simulink model "vllms_8_tap"  (R2021a)
settings: Solver=VariableStepAuto  StartTime=0.0  StopTime=4000  RelTol=1e-3
undefined symbols (not defined in the file): LeakyFactorCalc
libraries: dspsrcs4 x4, dspstat3 x4, dspmathops x2
settings Model: Creator=HP  LastModifiedBy=HP

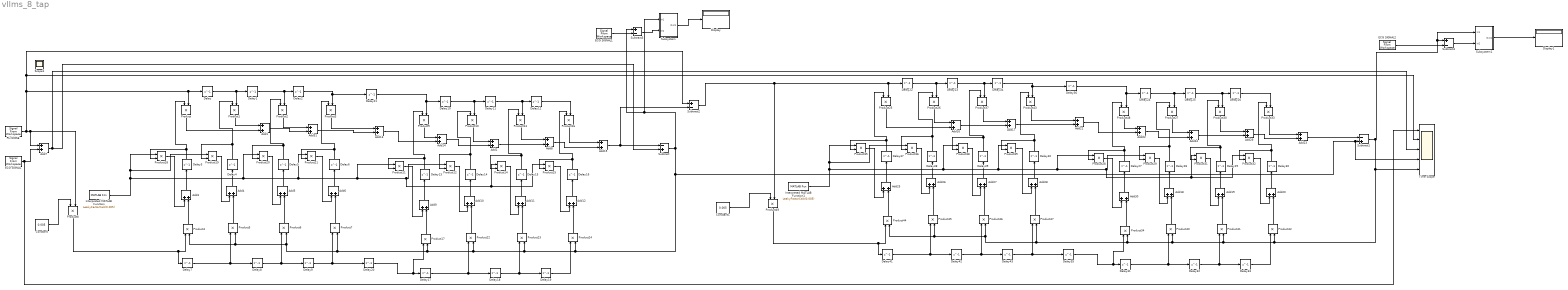
== system vllms_8_tap ==
  Add{1..31} (31 alike) : Sum
  Constant : Constant  Value=0.005
  Constant1 : Constant  Value=0.005
  Delay{,1..43} (44 alike) : Delay  DelayLength=1  InitialCondition=0
  Display : Display
  Display1 : Display
  ECG SIGNAL : dspsrcs4/Signal From Workspace  X=m1  Ts=1  nsamps=1  OutputAfterFinalValue=Setting to zero  ignoreOrWarnInputAndFrameLengths=off  OutputFrames=off
  ECG SIGNAL1 : dspsrcs4/Signal From Workspace  X=m1  Ts=1  nsamps=1  OutputAfterFinalValue=Setting to zero  ignoreOrWarnInputAndFrameLengths=off  OutputFrames=off
  ECG SIGNAL2 : dspsrcs4/Signal From Workspace  X=m1  Ts=1  nsamps=1  OutputAfterFinalValue=Setting to zero  ignoreOrWarnInputAndFrameLengths=off  OutputFrames=off
  Interpreted MATLAB Function : MATLABFcn  MATLABFcn=LeakyFactorCalc(0.005)
  Interpreted MATLAB Function1 : MATLABFcn  MATLABFcn=LeakyFactorCalc(0.005)
  PLI NOISE : dspsrcs4/Signal From Workspace  X=x1  Ts=1  nsamps=1  OutputAfterFinalValue=Setting to zero  ignoreOrWarnInputAndFrameLengths=off  OutputFrames=off
  Product{,1..49} (50 alike) : Product
  Subsystem : Subsystem
  Subsystem1 : Subsystem
  Subtract : Sum  Inputs=-+
  Subtract1 : Sum  Inputs=-+
  Subtract2 : Sum  Inputs=+-
  Subtract3 : Sum  Inputs=+-
  Subtract4 : Sum  Inputs=+-
  Time Scope : Scope  NumInputPorts=5
  Scope1 : Scope
  wires:
  Product7/1 -> Add6/2
  Delay6/1 -> Product21/2, Product3/1
  Delay1/1 -> Product2/2, Delay2/1
  PLI NOISE/1 -> Subtract2/1, Time Scope/2, Product/2, Delay/1, Product8/2, Add7/1
  Add4/1 -> Delay4/1
  Delay5/1 -> Product20/2, Product2/1
  Product5/1 -> Add4/2
  Product19/1 -> Add4/1
  Add5/1 -> Delay5/1
  Add6/1 -> Delay6/1
  Delay7/1 -> Delay8/1, Product5/1
  Product8/1 -> Product4/1, Delay7/1
  Delay8/1 -> Delay9/1, Product6/1
  Add3/1 -> Delay3/1
  Delay4/1 -> Product19/2, Product1/1
  Product4/1 -> Add3/2
  Product6/1 -> Add5/2
  Delay3/1 -> Product/1, Product18/2
  Product21/1 -> Add6/1
  Delay/1 -> Product1/2, Delay1/1
  Product20/1 -> Add5/1
  Product18/1 -> Add3/1
  Constant/1 -> Product8/1
  Product17/1 -> Add9/2
  Add9/1 -> Delay13/1
  Delay18/1 -> Delay19/1, Product23/1
  Delay11/1 -> Product13/2, Delay12/1
  Product24/1 -> Add12/2
  Interpreted MATLAB Function/1 -> Product20/1, Product21/1, Product14/1, Product15/1, Product12/1, Product11/1, Product19/1, Product18/1
  Add10/1 -> Delay14/1
  Product23/1 -> Add11/2
  Delay17/1 -> Delay18/1, Product22/1
  Delay12/1 -> Product16/2
  Product13/1 -> Add8/1
  Add12/1 -> Delay16/1
  Add2/1 -> Add8/2
  Add11/1 -> Delay15/1
  Delay9/1 -> Delay20/1, Product7/1
  Product12/1 -> Add10/1
  Product22/1 -> Add10/2
  Delay15/1 -> Product14/2, Product13/1
  Delay19/1 -> Product24/1
  Delay16/1 -> Product15/2, Product16/1
  Delay13/1 -> Product9/1, Product11/2
  Product15/1 -> Add12/1
  Product11/1 -> Add9/1
  Delay10/1 -> Product10/2, Delay11/1
  Delay14/1 -> Product12/2, Product10/1
  Product14/1 -> Add11/1
  Product10/1 -> Add2/1
  Delay2/1 -> Delay21/1, Product3/2
  Product9/1 -> Add14/1
  Add13/1 -> Add14/2
  Add14/1 -> Add2/2
  Add15/1 -> Subtract2/2, Subtract/1
  Product16/1 -> Add15/1
  Add8/1 -> Add15/2
  Delay20/1 -> Product17/1, Delay17/1
  Delay21/1 -> Product9/2, Delay10/1
  Add7/1 -> Time Scope/3, Subtract/2
  Add25/1 -> Delay37/1
  Product35/1 -> Add25/1
  Delay25/1 -> Product30/2, Delay26/1
  Product46/1 -> Add27/2
  Delay38/1 -> Product36/2, Product26/1
  Delay42/1 -> Delay43/1, Product46/1
  Product44/1 -> Add25/2
  Product43/1 -> Add21/1
  Delay28/1 -> Product29/2, Product27/1
  Delay29/1 -> Product31/2, Product30/1
  Subtract/1 -> Subsystem/1(In1), Subtract3/1, Time Scope/4, Subtract1/2, Product24/2, Product23/2, Product22/2, Product17/2, Product7/2, Product5/2, Product4/2, Product6/2
  Add26/1 -> Delay38/1
  Add29/1 -> Add23/2
  Delay34/1 -> Delay36/1, Product43/2
  Delay35/1 -> Product34/1, Delay31/1
  Product45/1 -> Add26/2
  Product31/1 -> Add19/1
  Add17/1 -> Add21/2
  Add27/1 -> Delay39/1
  Add18/1 -> Delay28/1
  Add20/1 -> Delay30/1
  Delay36/1 -> Product48/2, Delay24/1
  Delay27/1 -> Product48/1, Product28/2
  Delay22/1 -> Product26/2, Delay23/1
  Product26/1 -> Add16/1
  Add22/1 -> Add24/2
  Product34/1 -> Add30/2
  Product36/1 -> Add26/1
  Product41/1 -> Add19/2
  Product25/1 -> Add16/2
  Delay43/1 -> Delay35/1, Product47/1
  Add21/1 -> Add22/2
  Delay32/1 -> Delay33/1, Product41/1
  Product33/1 -> Add23/1
  Add23/1 -> Subtract1/1
  Product29/1 -> Add18/1
  Product28/1 -> Add30/1
  Delay24/1 -> Product27/2, Delay25/1
  Product38/1 -> Add27/1
  Delay37/1 -> Product25/1, Product35/2
  Delay30/1 -> Product32/2, Product33/1
  Product32/1 -> Add20/1
  Product42/1 -> Add20/2
  Add30/1 -> Delay27/1
  Subtract2/1 -> Product49/2, Product25/2, Delay22/1
  Interpreted MATLAB Function1/1 -> Product38/1, Product39/1, Product31/1, Product32/1, Product29/1, Product28/1, Product36/1, Product35/1
  Delay41/1 -> Delay42/1, Product45/1
  Add19/1 -> Delay29/1
  Product39/1 -> Add28/1
  Delay31/1 -> Delay32/1, Product40/1
  Add24/1 -> Add29/2
  Product30/1 -> Add29/1
  Product37/1 -> Add17/1
  Product40/1 -> Add18/2
  Delay40/1 -> Product39/2, Product43/1
  Delay39/1 -> Product38/2, Product37/1
  Add28/1 -> Delay40/1
  Product48/1 -> Add22/1
  Delay23/1 -> Product37/2, Delay34/1
  Product27/1 -> Add24/1
  Delay26/1 -> Product33/2
  Product49/1 -> Product44/1, Delay41/1
  Add16/1 -> Add17/2
  Product47/1 -> Add28/2
  Delay33/1 -> Product42/1
  Constant1/1 -> Product49/1
  ECG SIGNAL/1 -> Time Scope/1, Add7/2
  Subsystem/1(Out1) -> Display/1
  ECG SIGNAL1/1 -> Subtract3/2
  Subtract3/1 -> Subsystem/2(In2)
  Subtract4/1 -> Subsystem1/2(In2)
  Subsystem1/1(Out1) -> Display1/1
  ECG SIGNAL2/1 -> Subtract4/2
  Subtract1/1 -> Subsystem1/1(In1), Subtract4/1, Product42/2, Product41/2, Product40/2, Product34/2, Product47/2, Product45/2, Product44/2, Product46/2, Time Scope/5
  Product1/1 -> Add1/1
  Product/1 -> Add1/2
  Add1/1 -> Add31/2
  Product2/1 -> Add31/1
  Product3/1 -> Add13/1
  Add31/1 -> Add13/2

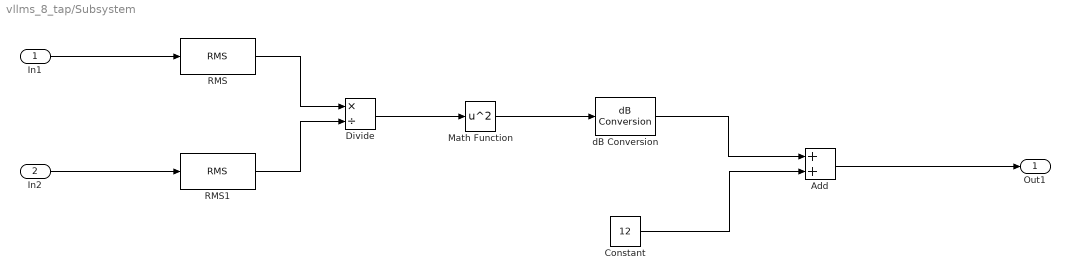
== system vllms_8_tap/Subsystem ==
  In1 : Inport
  In2 : Inport  Port=2
  Add : Sum
  Constant : Constant  Value=12
  Divide : Product  Inputs=*/
  Math Function : Math  Operator=square  SignedPower=on  OutputSignalType=real  SaturateOnIntegerOverflow=on
  RMS : dspstat3/RMS  run=on  directionMode=Each column  dimension=1  InputProcessing=Columns as channels (frame based)  reset_popup=None
  RMS1 : dspstat3/RMS  run=on  directionMode=Each column  dimension=1  InputProcessing=Columns as channels (frame based)  reset_popup=None
  dB Conversion : dspmathops/dB Conversion  dBtype=dB  intype=Amplitude  R=1  fuzz=off
  Out1 : Outport
  wires:
  RMS1/1 -> Divide/2
  dB Conversion/1 -> Add/1
  In1/1 -> RMS/1
  Divide/1 -> Math Function/1
  RMS/1 -> Divide/1
  In2/1 -> RMS1/1
  Add/1 -> Out1/1
  Constant/1 -> Add/2
  Math Function/1 -> dB Conversion/1

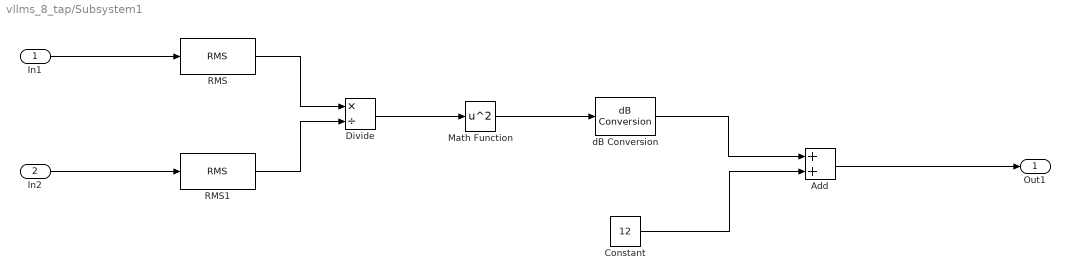
== system vllms_8_tap/Subsystem1 ==
  In1 : Inport
  In2 : Inport  Port=2
  Add : Sum
  Constant : Constant  Value=12
  Divide : Product  Inputs=*/
  Math Function : Math  Operator=square  SignedPower=on  OutputSignalType=real  SaturateOnIntegerOverflow=on
  RMS : dspstat3/RMS  run=on  directionMode=Each column  dimension=1  InputProcessing=Columns as channels (frame based)  reset_popup=None
  RMS1 : dspstat3/RMS  run=on  directionMode=Each column  dimension=1  InputProcessing=Columns as channels (frame based)  reset_popup=None
  dB Conversion : dspmathops/dB Conversion  dBtype=dB  intype=Amplitude  R=1  fuzz=off
  Out1 : Outport
  wires:
  RMS1/1 -> Divide/2
  dB Conversion/1 -> Add/1
  In1/1 -> RMS/1
  Divide/1 -> Math Function/1
  RMS/1 -> Divide/1
  In2/1 -> RMS1/1
  Add/1 -> Out1/1
  Constant/1 -> Add/2
  Math Function/1 -> dB Conversion/1
